simulink library "Copy_of_fluidDynamicSurface_cl_hydroelasticVersion"  (R2022a)
settings: Solver=VariableStepAuto  StartTime=0.0  StopTime=10.0  RelTol=1e-3
undefined symbols (not defined in the file or in its folder): env, vcl
libraries: calcFluidDynamicLoads x2, calcFluidDynamicLoads_hydroelasticVersion x2, eeGeneralControl x1
settings Model: Creator=mcobb  LastModifiedBy=Carson
settings SolverCC: AlgebraicLoopSolver=TrustRegion
settings DataIOCC: ReturnWorkspaceOutputs=off
settings DebuggingCC: UnconnectedInputMsg=warning  UnconnectedOutputMsg=warning  UnconnectedLineMsg=warning  SFMachineParentedDataDiag=warning  ArithmeticOperatorsInVariantConditions=warning
settings SFSimCC: CustomCodeUndefinedFunction=UseInterfaceOnly

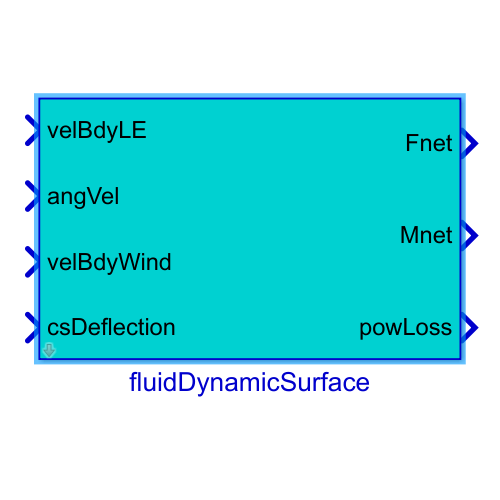
[thumbnail: Simulink's stored preview of the top-level diagram]
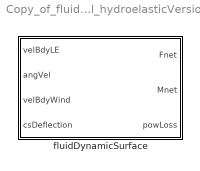
== system Copy_of_fluidDynamicSurface_cl_hydroelasticVersion ==
  fluidDynamicSurface : Subsystem  mask{vcl=vcl, fluidDensity=env.water.density.Value, fluidMomentArms=vcl.fluidMomentArms.Value, fluidRefArea=vcl.fluidRefArea.Value, wingTips=vcl.wingTipPositions.Value}
      mask prompts: vcl "Vehicle object"; fluidDensity "Fluid density"; fluidMomentArms "Fluid Moment Arms"; fluidRefArea "Fluid Reference Area"; wingTips "Wing Tips"
      mask help:
      | Input must be an 1×N struct array with fields:
      |     refArea
      |     aeroCentPosVec
      |     spanUnitVec
      |     chordUnitVec
      |     CL
      |     CD
      |     alpha
      |     GainCL
      |     GainCD
      |
      | where N is the number of aerodynamic surfaces
      settings: MinAlgLoopOccurrences=on

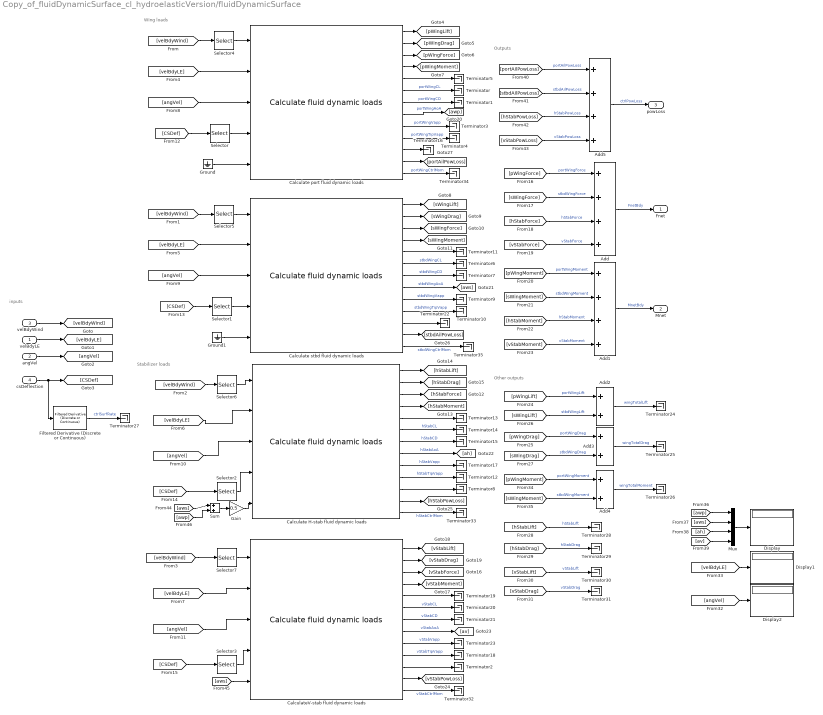
== system Copy_of_fluidDynamicSurface_cl_hydroelasticVersion/fluidDynamicSurface ==
  note: Other outputs
  note: Outputs
  note: WIng loads
  note: Stabilizer loads
  note: inputs
  velBdyLE : Inport
  angVel : Inport  Port=2
  velBdyWind : Inport  Port=3
  csDeflection : Inport  Port=4
  Add : Sum  Inputs=++++
  Add1 : Sum  Inputs=++++
  Add2 : Sum
  Add3 : Sum
  Add4 : Sum
  Add5 : Sum  Inputs=++++
  Calculate H-stab fluid dynamic loads : calcFluidDynamicLoads/Calculate fluid dynamic loads  aSurf=vcl.hStab  sRef=fluidRefArea  rArm_LE=fluidMomentArms(:,3)  rTip_LE=wingTips(:,3)  fluidDensity=fluidDensity
  Calculate port fluid dynamic loads : calcFluidDynamicLoads_hydroelasticVersion/Calculate fluid dynamic loads  aSurf=vcl.portWing  sRef=fluidRefArea  rArm_LE=fluidMomentArms(:,1)  rTip_LE=wingTips(:,1)  fluidDensity=fluidDensity
  Calculate stbd fluid dynamic loads : calcFluidDynamicLoads_hydroelasticVersion/Calculate fluid dynamic loads  aSurf=vcl.portWing  sRef=fluidRefArea  rArm_LE=fluidMomentArms(:,1)  rTip_LE=wingTips(:,1)  fluidDensity=fluidDensity
  CalculateV-stab fluid dynamic loads : calcFluidDynamicLoads/Calculate fluid dynamic loads  aSurf=vcl.vStab  sRef=fluidRefArea  rArm_LE=fluidMomentArms(:,4)  rTip_LE=wingTips(:,4)  fluidDensity=fluidDensity
  Display : Display
  Display1 : Display
  Display2 : Display
  Filtered Derivative (Discrete or Continuous) : eeGeneralControl/Filtered Derivative (Discrete or Continuous)  K=1  T=.001  B=inf  A=-inf  minRatio=10  init_option=Inherited from block input  x0=0  Ts=-1
      settings: SourceProductBaseCode=PS
  Gain : Gain  Gain=0.5
  Ground : Ground
  Ground1 : Ground
  Mux : Mux
  Selector : Selector  InputPortWidth=4  IndexOptions=Index vector (dialog)  Indices=1  OutputSizes=1
  Selector1 : Selector  InputPortWidth=4  IndexOptions=Index vector (dialog)  Indices=2  OutputSizes=1
  Selector2 : Selector  InputPortWidth=4  IndexOptions=Index vector (dialog)  Indices=3  OutputSizes=1
  Selector3 : Selector  InputPortWidth=4  IndexOptions=Index vector (dialog)  Indices=4  OutputSizes=1
  Selector4 : Selector  NumberOfDimensions=2  InputPortWidth=4  IndexOptions=Select all,Index vector (dialog)  Indices=1,1  OutputSizes=1,1
  Selector5 : Selector  NumberOfDimensions=2  InputPortWidth=4  IndexOptions=Select all,Index vector (dialog)  Indices=1,2  OutputSizes=1,1
  Selector6 : Selector  NumberOfDimensions=2  InputPortWidth=4  IndexOptions=Select all,Index vector (dialog)  Indices=1,3  OutputSizes=1,1
  Selector7 : Selector  NumberOfDimensions=2  InputPortWidth=4  IndexOptions=Select all,Index vector (dialog)  Indices=1,4  OutputSizes=1,1
  Sum : Sum  Inputs=|++
  Terminator{,1..35} (36 alike) : Terminator
  Fnet : Outport
  Mnet : Outport  Port=2
  powLoss : Outport  Port=3
  wires:
  angVel/1 -> [angVel]
  velBdyLE/1 -> [velBdyLE]
  velBdyWind/1 -> [velBdyWind]
  csDeflection/1 -> Filtered Derivative (Discrete or Continuous)/1, [CSDef]
  [velBdyWind] -> Selector4/1
  [velBdyWind] -> Selector5/1
  [velBdyWind] -> Selector6/1
  [velBdyWind] -> Selector7/1
  [velBdyLE] -> Calculate port fluid dynamic loads/2
  [velBdyLE] -> Calculate stbd fluid dynamic loads/2
  [velBdyLE] -> Calculate H-stab fluid dynamic loads/2
  [velBdyLE] -> CalculateV-stab fluid dynamic loads/2
  [angVel] -> Calculate port fluid dynamic loads/3
  [angVel] -> Calculate stbd fluid dynamic loads/3
  [angVel] -> Calculate H-stab fluid dynamic loads/3
  [angVel] -> CalculateV-stab fluid dynamic loads/3
  [CSDef] -> Selector/1
  Selector/1 -> Calculate port fluid dynamic loads/4
  Selector1/1 -> Calculate stbd fluid dynamic loads/4
  [CSDef] -> Selector1/1
  [CSDef] -> Selector2/1
  [CSDef] -> Selector3/1
  Selector2/1 -> Calculate H-stab fluid dynamic loads/4
  Selector3/1 -> CalculateV-stab fluid dynamic loads/4
  Calculate port fluid dynamic loads/1 -> [pWingLift]
  Calculate port fluid dynamic loads/2 -> [pWingDrag]
  Calculate port fluid dynamic loads/3 -> [pWingForce]
  Calculate port fluid dynamic loads/4 -> [pWingMoment]
  Calculate port fluid dynamic loads/6 -> Terminator/1  "portWingCL"
  Calculate port fluid dynamic loads/7 -> Terminator1/1  "portWingCD"
  Calculate port fluid dynamic loads/8 -> [awp]  "portWingAoA"
  Calculate port fluid dynamic loads/9 -> Terminator3/1  "portWingVapp"
  Calculate port fluid dynamic loads/10 -> Terminator4/1  "portWingTipVapp"
  Calculate port fluid dynamic loads/5 -> Terminator5/1
  Calculate stbd fluid dynamic loads/5 -> Terminator11/1
  Calculate stbd fluid dynamic loads/9 -> Terminator9/1  "stbdWingVapp"
  Calculate stbd fluid dynamic loads/6 -> Terminator6/1  "stbdWingCL"
  Calculate stbd fluid dynamic loads/8 -> [aws]  "stbdWingAoA"
  Calculate stbd fluid dynamic loads/7 -> Terminator7/1  "stbdWingCD"
  Calculate stbd fluid dynamic loads/10 -> Terminator10/1  "stbdWingTipVapp"
  Calculate stbd fluid dynamic loads/1 -> [sWingLift]
  Calculate stbd fluid dynamic loads/2 -> [sWingDrag]
  Calculate stbd fluid dynamic loads/3 -> [sWingForce]
  Calculate stbd fluid dynamic loads/4 -> [sWingMoment]
  Calculate H-stab fluid dynamic loads/2 -> [hStabDrag]
  Calculate H-stab fluid dynamic loads/4 -> [hStabMoment]
  Calculate H-stab fluid dynamic loads/5 -> Terminator13/1
  Calculate H-stab fluid dynamic loads/7 -> Terminator15/1  "hStabCD"
  Calculate H-stab fluid dynamic loads/1 -> [hStabLift]
  Calculate H-stab fluid dynamic loads/6 -> Terminator14/1  "hStabCL"
  Calculate H-stab fluid dynamic loads/3 -> [hStabForce]
  Calculate H-stab fluid dynamic loads/8 -> [ah]  "hStabAoA"
  Calculate H-stab fluid dynamic loads/10 -> Terminator12/1  "hStabTipVapp"
  Calculate H-stab fluid dynamic loads/9 -> Terminator17/1  "hStabVapp"
  CalculateV-stab fluid dynamic loads/3 -> [vStabForce]
  CalculateV-stab fluid dynamic loads/1 -> [vStabLift]
  CalculateV-stab fluid dynamic loads/6 -> Terminator20/1  "vStabCL"
  CalculateV-stab fluid dynamic loads/9 -> Terminator23/1  "vStabVapp"
  CalculateV-stab fluid dynamic loads/4 -> [vStabMoment]
  CalculateV-stab fluid dynamic loads/8 -> [av]  "vStabAoA"
  CalculateV-stab fluid dynamic loads/5 -> Terminator19/1
  CalculateV-stab fluid dynamic loads/2 -> [vStabDrag]
  CalculateV-stab fluid dynamic loads/10 -> Terminator18/1  "vStabTipVapp"
  CalculateV-stab fluid dynamic loads/7 -> Terminator21/1  "vStabCD"
  [pWingForce] -> Add/1  "portWingForce"
  [sWingForce] -> Add/2  "stbdWingForce"
  [vStabForce] -> Add/4  "vStabForce"
  [hStabForce] -> Add/3  "hStabForce"
  Add/1 -> Fnet/1  "FnetBdy"
  Add1/1 -> Mnet/1  "MnetBdy"
  [vStabMoment] -> Add1/4  "vStabMoment"
  [hStabMoment] -> Add1/3  "hStabMoment"
  [sWingMoment] -> Add1/2  "stbdWingMoment"
  [pWingMoment] -> Add1/1  "portWingMoment"
  [vStabDrag] -> Terminator31/1  "vStabDrag"
  [vStabLift] -> Terminator30/1  "vStabLift"
  [hStabDrag] -> Terminator29/1  "hStabDrag"
  [hStabLift] -> Terminator28/1  "hStabLift"
  [sWingDrag] -> Add3/2  "stbdWingDrag"
  [sWingLift] -> Add2/2  "stbdWingLift"
  [pWingDrag] -> Add3/1  "portWingDrag"
  [pWingLift] -> Add2/1  "portWingLift"
  Selector4/1 -> Calculate port fluid dynamic loads/1
  Selector5/1 -> Calculate stbd fluid dynamic loads/1
  Selector6/1 -> Calculate H-stab fluid dynamic loads/1
  Selector7/1 -> CalculateV-stab fluid dynamic loads/1
  Add2/1 -> Terminator24/1  "wingTotalLift"
  Add3/1 -> Terminator25/1  "wingTotalDrag"
  Add4/1 -> Terminator26/1  "wingTotalMoment"
  [pWingMoment] -> Add4/1  "portWingMoment"
  [sWingMoment] -> Add4/2  "stbdWingMoment"
  [av] -> Mux/4
  [ah] -> Mux/3
  [aws] -> Mux/2
  [awp] -> Mux/1
  Mux/1 -> Display/1
  [angVel] -> Display2/1
  [velBdyLE] -> Display1/1
  Calculate port fluid dynamic loads/11 -> Terminator16/1
  Calculate stbd fluid dynamic loads/11 -> Terminator22/1
  Calculate H-stab fluid dynamic loads/11 -> Terminator8/1
  CalculateV-stab fluid dynamic loads/11 -> Terminator2/1
  CalculateV-stab fluid dynamic loads/12 -> [vStabPowLoss]
  Calculate H-stab fluid dynamic loads/12 -> [hStabPowLoss]
  Calculate stbd fluid dynamic loads/12 -> [stbdAilPowLoss]
  Calculate port fluid dynamic loads/12 -> [portAilPowLoss]
  [portAilPowLoss] -> Add5/1  "portAilPowLoss"
  [stbdAilPowLoss] -> Add5/2  "stbdAilPowLoss"
  Add5/1 -> powLoss/1  "ctrlPowLoss"
  [hStabPowLoss] -> Add5/3  "hStabPowLoss"
  [vStabPowLoss] -> Add5/4  "vStabPowLoss"
  Filtered Derivative (Discrete or Continuous)/1 -> Terminator27/1  "ctrlSurfRate"
  CalculateV-stab fluid dynamic loads/13 -> Terminator32/1  "vStabCtrlMom"
  Calculate H-stab fluid dynamic loads/13 -> Terminator33/1  "hStabCtrlMom"
  Calculate port fluid dynamic loads/13 -> Terminator34/1  "portWingCtrlMom"
  Calculate stbd fluid dynamic loads/13 -> Terminator35/1  "stbdWingCtrlMom"
  [aws] -> CalculateV-stab fluid dynamic loads/5
  [aws] -> Sum/1
  [awp] -> Sum/2
  Gain/1 -> Calculate H-stab fluid dynamic loads/5
  Sum/1 -> Gain/1
  Ground/1 -> Calculate port fluid dynamic loads/5
  Ground1/1 -> Calculate stbd fluid dynamic loads/5
